simulink model "doc_crcgen"  (R2014a)
settings: Solver=FixedStepDiscrete  SolverMode=SingleTasking  StartTime=0.0  StopTime=6  RelTol=1e-3
PreLoadFcn:
  | iniStates = [ 0 1 1];
undefined symbols (not defined in the file or in its folder): commblksprivate, Info
libraries: commcrc2 x1, dspsrcs4 x1, dspsigops x1
settings Model: Creator=The MathWorks Inc.
settings DataIOCC: SignalLoggingSaveFormat=ModelDataLogs
settings OptimizationCC: ExpressionDepthLimit=2147483647  InitFltsAndDblsToZero=on
settings DebuggingCC: SaveWithParameterizedLinksMsg=none  UnderspecifiedInitializationDetection=Classic  SignalResolutionControl=TryResolveAllWithWarning  FcnCallInpInsideContextMsg=UseLocalSettings  StateNameClashWarn=warning  StrictBusMsg=Warning
settings GRTTargetCC: TargetFcnLib=ansi_tfl_tmw.mat  CombineOutputUpdateFcns=off  GRTInterface=on

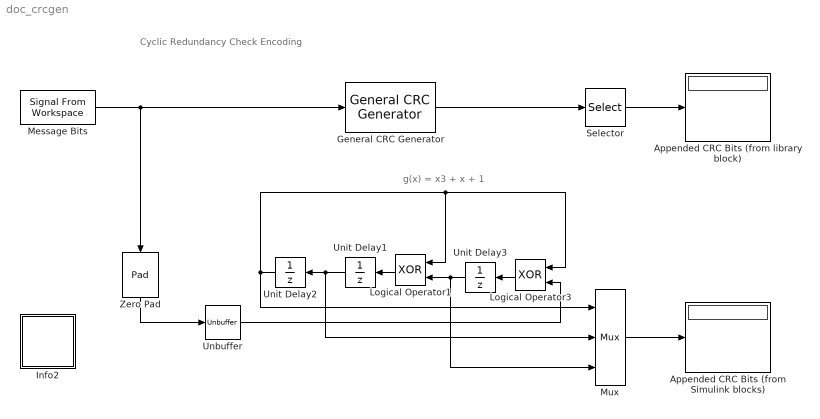
== system doc_crcgen ==
  note: g(x) = x3 + x + 1
  note: Cyclic Redundancy Check Encoding
  Appended CRC Bits (from Simulink blocks) : Display
  Appended CRC Bits (from library block) : Display
  General CRC Generator : commcrc2/General CRC Generator  genPoly=[1 0 1 1]  iniStates=iniStates  directMethod=off  reflectInputBytes=off  reflectChecksums=off  finalXOR=0  numChecksums=1
  Info2 : Subsystem  AncestorBlock=commblksprivate/Info  mask(Info){}
      settings: OpenFcn=helpview([docroot '/toolbox/comm/comm.map'], 'doc_crcgen')
      mask Display: disp('Info')
  Logical Operator1 : Logic  Operator=XOR  AllPortsSameDT=off  OutDataTypeStr=float('double')
  Logical Operator3 : Logic  Operator=XOR  AllPortsSameDT=off  OutDataTypeStr=float('double')
  Message Bits : dspsrcs4/Signal From Workspace  X=[1 1 1 0 1 0]  Ts=1  nsamps=6  OutputAfterFinalValue=Cyclic repetition  ignoreOrWarnInputAndFrameLengths=off
  Mux : Mux  Inputs=3
  Selector : Selector  InputPortWidth=9  Indices=[7:9]
  Unbuffer : Unbuffer  SampleBasedProcessing=Same as frame based
  Unit Delay1 : UnitDelay  InitialCondition=iniStates(2)  SampleTime=-1
  Unit Delay2 : UnitDelay  InitialCondition=iniStates(1)  SampleTime=-1
  Unit Delay3 : UnitDelay  InitialCondition=iniStates(3)  SampleTime=-1
  Zero Pad : dspsigops/Pad  padAlong=Columns  dimsToPad=1  valSrc=Specify via dialog  padVal=0  spec=Output size  padNumOutRowsSpecMethod=User-specified  numOutRows=6+3  padNumOutColsSpecMethod=User-specified  numOutCols=1  isVarDimsMode=off  padBeginning=0  padEnd=0  outSizeMode=User-specified  outSize=1  padSigAt=End  trunc_flag=None  roundingMode=Floor  overflowMode=off  truncOrWrapMode=Truncate  wrap_flag=None
  wires:
  Message Bits/1 -> General CRC Generator/1, Zero Pad/1
  General CRC Generator/1 -> Selector/1
  Unbuffer/1 -> Logical Operator3/2
  Zero Pad/1 -> Unbuffer/1
  Unit Delay1/1 -> Unit Delay2/1, Mux/2
  Unit Delay2/1 -> Logical Operator3/1, Logical Operator1/1, Mux/1
  Logical Operator1/1 -> Unit Delay1/1
  Unit Delay3/1 -> Logical Operator1/2, Mux/3
  Logical Operator3/1 -> Unit Delay3/1
  Mux/1 -> Appended CRC Bits (from Simulink blocks)/1
  Selector/1 -> Appended CRC Bits (from library block)/1

== system doc_crcgen/Info2 ==
